simulink model "Half_Band_Filter_fc500_fs4k"  (R2022b)
settings: Solver=FixedStepAuto  StartTime=0.0  StopTime=1  FixedStep=1/4000  RelTol=1e-3
model workspace (MAT data in the model file):
  TS = 0.00025
settings Model: Creator=Rio  LastModifiedBy=Rio
settings DebuggingCC: ParameterPrecisionLossMsg=none

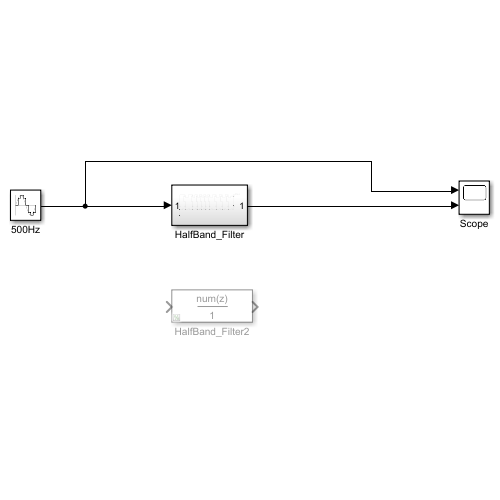
[thumbnail: Simulink's stored preview of the top-level diagram]
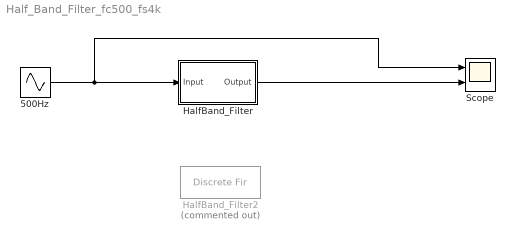
== system Half_Band_Filter_fc500_fs4k ==
  500Hz : Sin  Frequency=2*pi*400  SampleTime=TS
  HalfBand_Filter : Subsystem  Tag=FilterWizardSubSystem
      settings: ErrorFcn=dspFilterRealizedInBasicElemsAlgLoopErrFcnCallback
  HalfBand_Filter2 : DiscreteFir  Tag=BlockMethodSubSystem  Commented=on  Coefficients=[0.00112238603488490352 0 -0.00711382316853739934 0 0.0262000101640785799 0 -0.0779544398789242948 0 0.307764312260402184 0.5 0.307764312260402184 0 -0.0779544398789242948 0 0.0262000101640785799 0 -0.00711382316853739934 0 0.00112238603488490352]  InputProcessing=Columns as channels (frame based)
  Scope : Scope  NumInputPorts=2
  wires:
  500Hz/1 -> Scope/1, HalfBand_Filter/1(Input)
  HalfBand_Filter/1(Output) -> Scope/2

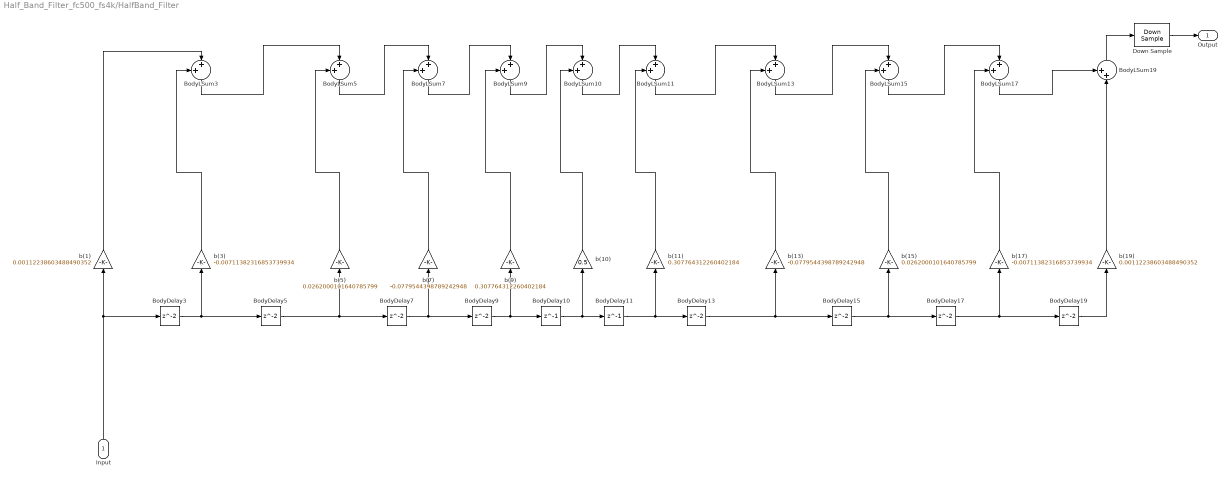
== system Half_Band_Filter_fc500_fs4k/HalfBand_Filter ==
  Input : Inport
  BodyDelay10 : Delay  DelayLength=1  InitialCondition=0  InputProcessing=Columns as channels (frame based)
  BodyDelay11 : Delay  DelayLength=1  InitialCondition=0  InputProcessing=Columns as channels (frame based)
  BodyDelay{3,5,7,9,13,15,17,19} (8 alike) : Delay  InitialCondition=0  InputProcessing=Columns as channels (frame based)
  BodyLSum{3,5,7,9..11,13,15,17,19} (10 alike) : Sum  Inputs=++|  RndMeth=Nearest  SaturateOnIntegerOverflow=on  OutDataTypeStr=Inherit: Same as first input
  Down Sample : DownSample  RateOptions=Allow multirate processing  AllowArbitraryFixedInput=on
  b(1) : Gain  Gain=0.00112238603488490352  ParamDataTypeStr=single  RndMeth=Nearest  SaturateOnIntegerOverflow=on  OutDataTypeStr=Inherit: Same as input
  b(10) : Gain  Gain=0.5  ParamDataTypeStr=single  RndMeth=Nearest  SaturateOnIntegerOverflow=on  OutDataTypeStr=Inherit: Same as input
  b(11) : Gain  Gain=0.307764312260402184  ParamDataTypeStr=single  RndMeth=Nearest  SaturateOnIntegerOverflow=on  OutDataTypeStr=Inherit: Same as input
  b(13) : Gain  Gain=-0.0779544398789242948  ParamDataTypeStr=single  RndMeth=Nearest  SaturateOnIntegerOverflow=on  OutDataTypeStr=Inherit: Same as input
  b(15) : Gain  Gain=0.0262000101640785799  ParamDataTypeStr=single  RndMeth=Nearest  SaturateOnIntegerOverflow=on  OutDataTypeStr=Inherit: Same as input
  b(17) : Gain  Gain=-0.00711382316853739934  ParamDataTypeStr=single  RndMeth=Nearest  SaturateOnIntegerOverflow=on  OutDataTypeStr=Inherit: Same as input
  b(19) : Gain  Gain=0.00112238603488490352  ParamDataTypeStr=single  RndMeth=Nearest  SaturateOnIntegerOverflow=on  OutDataTypeStr=Inherit: Same as input
  b(3) : Gain  Gain=-0.00711382316853739934  ParamDataTypeStr=single  RndMeth=Nearest  SaturateOnIntegerOverflow=on  OutDataTypeStr=Inherit: Same as input
  b(5) : Gain  Gain=0.0262000101640785799  ParamDataTypeStr=single  RndMeth=Nearest  SaturateOnIntegerOverflow=on  OutDataTypeStr=Inherit: Same as input
  b(7) : Gain  Gain=-0.0779544398789242948  ParamDataTypeStr=single  RndMeth=Nearest  SaturateOnIntegerOverflow=on  OutDataTypeStr=Inherit: Same as input
  b(9) : Gain  Gain=0.307764312260402184  ParamDataTypeStr=single  RndMeth=Nearest  SaturateOnIntegerOverflow=on  OutDataTypeStr=Inherit: Same as input
  Output : Outport
  wires:
  Input/1 -> b(1)/1, BodyDelay3/1
  b(1)/1 -> BodyLSum3/2
  BodyDelay3/1 -> b(3)/1, BodyDelay5/1
  b(3)/1 -> BodyLSum3/1
  BodyLSum3/1 -> BodyLSum5/2
  BodyDelay5/1 -> b(5)/1, BodyDelay7/1
  b(5)/1 -> BodyLSum5/1
  BodyLSum5/1 -> BodyLSum7/2
  BodyDelay7/1 -> b(7)/1, BodyDelay9/1
  b(7)/1 -> BodyLSum7/1
  BodyLSum7/1 -> BodyLSum9/2
  BodyDelay9/1 -> b(9)/1, BodyDelay10/1
  b(9)/1 -> BodyLSum9/1
  BodyLSum9/1 -> BodyLSum10/2
  BodyDelay10/1 -> b(10)/1, BodyDelay11/1
  b(10)/1 -> BodyLSum10/1
  BodyLSum10/1 -> BodyLSum11/2
  BodyDelay11/1 -> b(11)/1, BodyDelay13/1
  b(11)/1 -> BodyLSum11/1
  BodyLSum11/1 -> BodyLSum13/2
  BodyDelay13/1 -> b(13)/1, BodyDelay15/1
  b(13)/1 -> BodyLSum13/1
  BodyLSum13/1 -> BodyLSum15/2
  BodyDelay15/1 -> b(15)/1, BodyDelay17/1
  b(15)/1 -> BodyLSum15/1
  BodyLSum15/1 -> BodyLSum17/2
  BodyDelay17/1 -> b(17)/1, BodyDelay19/1
  b(17)/1 -> BodyLSum17/1
  BodyLSum17/1 -> BodyLSum19/1
  BodyDelay19/1 -> b(19)/1
  b(19)/1 -> BodyLSum19/2
  BodyLSum19/1 -> Down Sample/1
  Down Sample/1 -> Output/1
